simulink model "test_case_generation_SOC"  (R2015b)
settings: Solver=FixedStepDiscrete  StartTime=0.0  StopTime=final_time  FixedStep=0.1  RelTol=1e-3
values from neighbouring files (symbols this model uses):
  BMSk_stepSize = 0.1    [soc_test_case_init.m]
  cell_ocvs_sampling = sampling_time    (= 0.1)    [soc_test_case_init.m]
  cell_socs_sampling = sampling_time    (= 0.1)    [soc_test_case_init.m]
  cell_temps_sampling = sampling_time    (= 0.1)    [soc_test_case_init.m]
  cell_voltages_sampling = sampling_time    (= 0.1)    [soc_test_case_init.m]
  charge_cycle = 4    [soc_test_case_init.m]
  inital_outlet_temperature = air_temperature    (= 35)    [soc_test_case_init.m]
  initial_cell_ocvs = Initial_Volt*ones(NUM_CELL_SERIES,1)    [soc_test_case_init.m]
  initial_cell_socs = Initial_SOC*ones(NUM_CELL_SERIES,1)    [soc_test_case_init.m]
  initial_cell_temps = air_temperature*ones(NUM_CELL_SERIES,1)    [soc_test_case_init.m]
  initial_cell_voltages = Initial_Volt*ones(NUM_CELL_SERIES,1)    [soc_test_case_init.m]
  initial_pack_current = 0    [soc_test_case_init.m]
  initial_pack_soc = Initial_SOC    (= 79)    [soc_test_case_init.m]
  initial_pack_voltage = 161    [soc_test_case_init.m]
  initial_vehicle_side_voltage = 0    [soc_test_case_init.m]
  pack_current_sampling = sampling_time    (= 0.1)    [soc_test_case_init.m]
  pack_soc_sampling = sampling_time    (= 0.1)    [soc_test_case_init.m]
  pack_voltage_sampling = sampling_time    (= 0.1)    [soc_test_case_init.m]
  vehicle_side_voltage_sampling = sampling_time    (= 0.1)    [soc_test_case_init.m]
undefined symbols (not defined in the file or in its folder): sigbuilder_block
libraries: simulink x4
(part 1 of 2)
settings Model: Creator=nctzv8  LastModifiedBy=nctzv8
settings ConfigSet: Description=OpenECU configuration set for code generation under RTW-EC.
settings SolverCC: PositivePriorityOrder=on
settings DataIOCC: SaveFormat=Array  SignalLoggingSaveFormat=ModelDataLogs
settings OptimizationCC: DefaultParameterBehavior=Inlined  InlineInvariantSignals=on  ExpressionDepthLimit=2147483647  StateBitsets=on  DataBitsets=on  ZeroExternalMemoryAtStartup=off  ZeroInternalMemoryAtStartup=off  NoFixptDivByZeroProtection=on  EfficientFloat2IntCast=on  OptimizeModelRefInitCode=on  LifeSpan=1
settings DebuggingCC: SaveWithParameterizedLinksMsg=none  UnderspecifiedInitializationDetection=Classic  MergeDetectMultiDrivingBlocksExec=none  SignalResolutionControl=TryResolveAllWithWarning  MultiTaskDSMMsg=warning  MultiTaskCondExecSysMsg=none  SingleTaskRateTransMsg=error  CheckMatrixSingularityMsg=warning  VectorMatrixConversionMsg=warning  FcnCallInpInsideContextMsg=UseLocalSettings  SignalLabelMismatchMsg=warning  StateNameClashWarn=warning
settings HardwareCC: ProdBitPerPointer=32  ProdLargestAtomicInteger=Long  ProdLargestAtomicFloat=Double  ProdEndianess=BigEndian  ProdWordSize=32  ProdHWDeviceType=Freescale->32-bit PowerPC  TargetIntDivRoundTo=Zero  TargetEndianess=BigEndian  TargetHWDeviceType=Freescale->32-bit PowerPC  ProdEqTarget=off
settings RTWCC: SystemTargetFile=openecu_ert.tlc  MakeCommand=make_rtw optimized_floating_point=1  TemplateMakefile=openecu_ert_r2015b_64.tmf  Description=OpenECU Platform Target (ERT, optimised floating-point code)  RetainRTWFile=on  IncludeHyperlinkInReport=on
settings CodeAppCC: ForceParamTrailComments=on  IgnoreCustomStorageClasses=off  SimulinkDataObjDesc=on  CustomSymbolStrType=$N$R$M  InsertBlockDesc=on  InternalIdentifier=Classic
settings STFCustomTargetCC: TargetLibSuffix=.a  GenerateSampleERTMain=on  ConcurrentExecutionCompliant=off  IncludeMdlTerminateFcn=off  GeneratePreprocessorConditionals=Use local settings  CombineOutputUpdateFcns=on  IncludeFileDelimiter=UseQuote  ERTCustomFileBanners=on  SupportContinuousTime=off  MATLABClassNameForMDSCustomization=Simulink.SoftwareTarget.ERTCustomization  CPPClassGenCompliant=off  GRTInterface=off  SystemTargetFile=openecu_ert.tlc
settings ERTTargetCC: GenerateSampleERTMain=on  ParMdlRefBuildCompliant=off  CompOptLevelCompliant=off  ConcurrentExecutionCompliant=off  IncludeMdlTerminateFcn=off  ERTFirstTimeCompliant=off  IncludeFileDelimiter=UseQuote  SupportNonInlinedSFcns=on  ModelStepFunctionPrototypeControlCompliant=off  CPPClassGenCompliant=off  UseToolchainInfoCompliant=off  ExtModeMexFile=noextcomm  InlinedParameterPlacement=NonHierarchical  ERTSrcFileBannerTemplate=oe_code_c_template.cgt  ERTHdrFileBannerTemplate=oe_code_h_template.cgt  ERTDataSrcFileTemplate=oe_data_c_template.cgt  ERTDataHdrFileTemplate=oe_data_h_template.cgt  ERTCustomFileTemplate=example_file_process.tlc  GlobalDataDefinition=InSeparateSourceFile  GlobalDataReference=InSeparateHeaderFile  EnableUserReplacementTypes=on

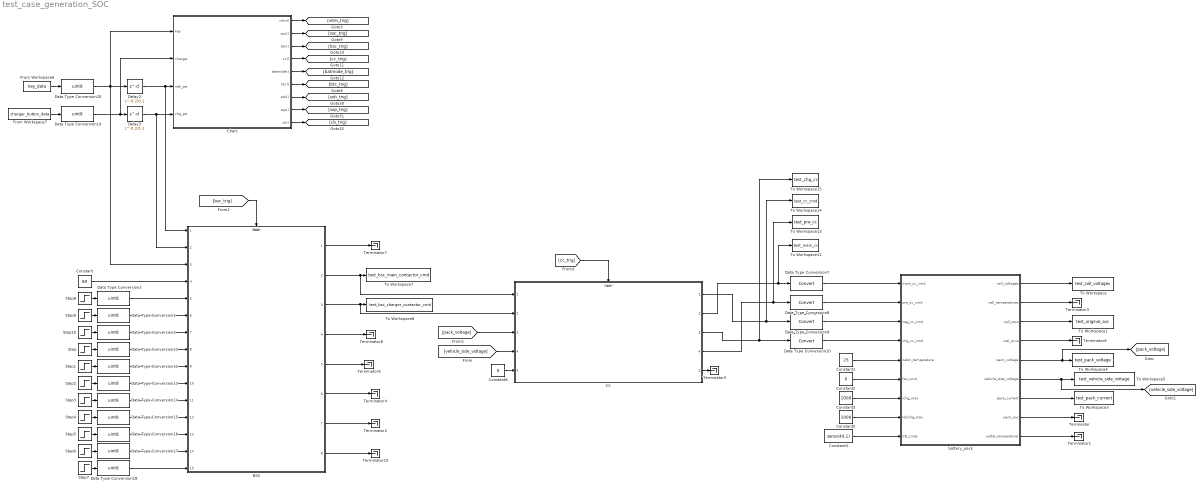
== system test_case_generation_SOC ==
  BSC : ModelReference  ModelNameDialog=BSC.slx  SimulationMode=Normal  ModelReferenceVersion=1.220  CopyOfModelName=BSC.slx  TriggerPortName=Trigger  TriggerPortTriggerType=function-call  TriggerPortStatesWhenEnabling=held
  CC : ModelReference  ModelNameDialog=CC.slx  SimulationMode=Normal  ModelReferenceVersion=1.108  CopyOfModelName=CC.slx  TriggerPortName=Trigger  TriggerPortTriggerType=function-call  TriggerPortStatesWhenEnabling=held
  Chart : Stateflow chart  TreatAsAtomicUnit=on
  Constant : Constant  Value=80
  Constant1 : Constant  Value=25
  Constant2 : Constant  Value=0
  Constant3 : Constant  Value=1000
  Constant4 : Constant  Value=zeros(40,1)
  Constant5 : Constant  Value=1000
  Constant6 : Constant  Value=0
  Data Type Conversion{1..3,11..20} (13 alike) : DataTypeConversion  OutDataTypeStr=uint8
  Data Type Conversion{7..10} (4 alike) : DataTypeConversion
  Delay2 : Delay  DelayLength=0.2/0.1
  Delay3 : Delay  DelayLength=0.2/0.1
  From Workspace6 : FromWorkspace  VariableName=key_data
  From Workspace7 : FromWorkspace  VariableName=charger_button_data
  Step{,1..10} (11 alike) : Step  Time=0  After=0  VectorParams1D=off
  Terminator{,1..10} (11 alike) : Terminator
  To Workspace : ToWorkspace  VariableName=test_cell_voltages  SaveFormat=Timeseries  SampleTime=-1
  To Workspace1 : ToWorkspace  VariableName=test_original_soc  SaveFormat=Timeseries  SampleTime=-1
  To Workspace12 : ToWorkspace  VariableName=test_main_cc  SaveFormat=Timeseries  SampleTime=-1
  To Workspace13 : ToWorkspace  VariableName=test_pre_cc  SaveFormat=Timeseries  SampleTime=-1
  To Workspace14 : ToWorkspace  VariableName=test_cc_cmd  SaveFormat=Timeseries  SampleTime=-1
  To Workspace15 : ToWorkspace  VariableName=test_chg_cc  SaveFormat=Timeseries  SampleTime=-1
  To Workspace3 : ToWorkspace  VariableName=test_pack_current  SaveFormat=Timeseries  SampleTime=-1
  To Workspace4 : ToWorkspace  VariableName=test_pack_voltage  SaveFormat=Timeseries  SampleTime=-1
  To Workspace5 : ToWorkspace  VariableName=test_vehicle_side_voltage  SaveFormat=Timeseries  SampleTime=-1
  To Workspace7 : ToWorkspace  VariableName=test_bsc_main_contactor_cmd  SaveFormat=Timeseries  SampleTime=-1
  To Workspace8 : ToWorkspace  VariableName=test_bsc_charger_contactor_cmd  SaveFormat=Timeseries  SampleTime=-1
  battery_pack : Subsystem
  wires:
  battery_pack/1(cell_voltages) -> To Workspace/1
  battery_pack/2(cell_temperatures) -> Terminator3/1
  battery_pack/3(cell_socs) -> To Workspace1/1
  battery_pack/4(cell_ocvs) -> Terminator6/1
  battery_pack/5(pack_voltage) -> [pack_voltage], To Workspace4/1
  battery_pack/6(vehicle_side_voltage) -> [vehicle_side_voltage], To Workspace5/1
  battery_pack/7(pack_current) -> To Workspace3/1
  battery_pack/8(pack_soc) -> Terminator/1
  battery_pack/9(outlet_temperature) -> Terminator1/1
  Constant1/1 -> battery_pack/5(cabin_temperature)
  Constant2/1 -> battery_pack/6(fan_cmd)
  Constant3/1 -> battery_pack/7(Ichg_max)
  Constant4/1 -> battery_pack/9(CB_cmds)
  Constant5/1 -> battery_pack/8(Idischg_max)
  Data Type Conversion7/1 -> battery_pack/1(main_cc_cmd)
  Data Type Conversion8/1 -> battery_pack/2(pre_cc_cmd)
  Data Type Conversion10/1 -> battery_pack/4(chg_cc_cmd)
  CC/1 -> To Workspace14/1, Data Type Conversion9/1
  CC/2 -> To Workspace12/1, Data Type Conversion7/1
  CC/3 -> To Workspace15/1, Data Type Conversion10/1
  CC/4 -> To Workspace13/1, Data Type Conversion8/1
  Constant/1 -> BSC/4
  Data Type Conversion2/1 -> BSC/5
  Data Type Conversion1/1 -> BSC/6
  Data Type Conversion3/1 -> BSC/7
  Data Type Conversion12/1 -> BSC/8
  Data Type Conversion13/1 -> BSC/10
  Data Type Conversion11/1 -> BSC/9
  Data Type Conversion14/1 -> BSC/11
  Data Type Conversion15/1 -> BSC/12
  Data Type Conversion17/1 -> BSC/14
  Data Type Conversion18/1 -> BSC/15
  Data Type Conversion16/1 -> BSC/13
  [bsc_trig] -> BSC/Trigger
  BSC/1 -> Terminator7/1
  BSC/2 -> CC/1, To Workspace7/1
  BSC/3 -> CC/2, To Workspace8/1
  BSC/4 -> Terminator8/1
  BSC/5 -> Terminator9/1
  BSC/7 -> Terminator2/1
  BSC/6 -> Terminator4/1
  BSC/8 -> Terminator10/1
  [vehicle_side_voltage] -> CC/4
  [pack_voltage] -> CC/3
  Constant6/1 -> CC/5
  [cc_trig] -> CC/Trigger
  Data Type Conversion9/1 -> battery_pack/3(neg_cc_cmd)
  CC/5 -> Terminator5/1
  Step2/1 -> Data Type Conversion13/1
  Step1/1 -> Data Type Conversion11/1
  Step3/1 -> Data Type Conversion14/1
  Step4/1 -> Data Type Conversion15/1
  Step6/1 -> Data Type Conversion17/1
  Step7/1 -> Data Type Conversion18/1
  Step5/1 -> Data Type Conversion16/1
  Step/1 -> Data Type Conversion12/1
  Step10/1 -> Data Type Conversion3/1
  Step9/1 -> Data Type Conversion1/1
  Step8/1 -> Data Type Conversion2/1
  Chart/1(vitm()) -> [vitm_trig]
  Chart/2(soc()) -> [soc_trig]
  Chart/3(bsc()) -> [bsc_trig]
  Chart/4(cc()) -> [cc_trig]
  Chart/5(batmode()) -> [batmode_trig]
  Chart/6(btc()) -> [btc_trig]
  Delay2/1 -> BSC/1, Chart/3(veh_psr)
  Chart/7(soh()) -> [soh_trig]
  Chart/8(sop()) -> [sop_trig]
  Chart/9(cb()) -> [cb_trig]
  Delay3/1 -> BSC/2, Chart/4(chg_psr)
  Data Type Conversion19/1 -> Chart/2(charger), Delay3/1
  Data Type Conversion20/1 -> BSC/3, Chart/1(key), Delay2/1
  From Workspace6/1 -> Data Type Conversion20/1
  From Workspace7/1 -> Data Type Conversion19/1

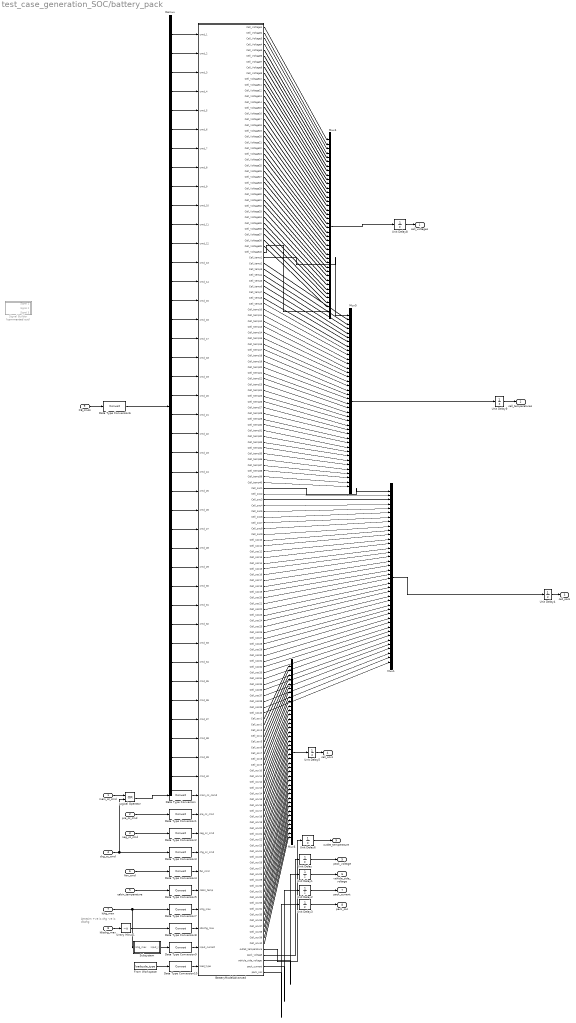
== system test_case_generation_SOC/battery_pack ==
  note: Amesim
      | +ve is chg
      | -ve is dischg
  main_cc_cmd : Inport
  pre_cc_cmd : Inport  Port=2
  neg_cc_cmd : Inport  Port=3
  chg_cc_cmd : Inport  Port=4
  cabin_temperature : Inport  Port=5
  fan_cmd : Inport  Port=6
  Ichg_max : Inport  Port=7
  Idischg_max : Inport  Port=8
  CB_cmds : Inport  Port=9
  BatteryModelAdvanced : Subsystem  Tag=AME2SLCoSim  InitFcn=AMESimLib_initBlock  StartFcn=AMESimLib_startBlock  StopFcn=AMESimLib_stopBlock
      settings: DeleteFcn=AMESimLib_deleteBlock  OpenFcn=AMESimLib_openBlock('AME2SLCoSim')
      mask Display: image(imread('amesim_pix256.png'),[0.4,0.7,0.2,0.2]);disp('Simcenter Amesim co-Sim:\nBatteryModelAdvanced');port_label('input',1,'cmd_1');port_label('input',2,'cmd_2');port_label('input',3,'cmd_3');port_label('input',4,'cmd_4');port_label('input',5,'cmd_5');port_label('input',6,'cmd_6');port_label('input',7,'cmd_7');port_label('input',8,'cmd_8');port_label('input',9,'cmd_9');port_label('input',10,'cmd_10');port_label('input',11,'cmd_11');port_label('input',12,'cmd_12');port_label('input',13,'cmd_13');port_label('input',14,'cmd_14');port_label('input',15,'cmd_15');port_label('input',16,'cmd_16');port_label('input',17,'cmd_17');port_label('input',18,'cmd_18');port_label('input',19,'cmd_19');port_label('input',20,'cmd_20');port_label('input',21,'cmd_21');port_label('input',22,'cmd_22');port_label('input',23,'cmd_23');port_label('input',24,'cmd_24');port_label('input',25,'cmd_25');port_label('input',26,'cmd_26');port_label('input',27,'cmd_27');port_label('input',28,'cmd_28');port_label('input',29,'cmd_29');port_label('input',30,'cmd_30');port_label('input',31,'cmd_31');port_label('input',32,'cmd_32');port_label('input',33,'cmd_33');port_label('input',34,'cmd_34');port_label('input',35,'cmd_35');port_label('input',36,'cmd_36');port_label('input',37,'cmd_37');port_label('input',38,'cmd_38');port_label('input',39,'cmd_39');port_label('input',40,'cmd_40');port_label('input',41,'main_cc_comd');port_label('input',42,'pre_cc_cmd');port_label('input',43,'neg_cc_cmd');port_label('input',44,'chg_cc_cmd');port_label('input',45,'fan_cmd');port_label('input',46,'cabin_temp');port_label('input',47,'Ichg_max');port_label('input',48,'Idischg_max');port_label('input',49,'input_current');port_label('input',50,'load_type');port_label('output',1,'Cell_Voltage1');port_label('output',2,'Cell_Voltage2');port_label('output',3,'Cell_Voltage3');port_label('output',4,'Cell_Voltage4');port_label('output',5,'Cell_Voltage5');port_label('output',6,'Cell_Voltage6');port_label('output',7,'Cell_Voltage7');port_label('output',8,'Cell_Voltage8');port_label('output',9,'Cell_Voltage9');port_label('output',10,'Cell_Voltage10');port_label('output',11,'Cell_Voltage11');port_label('output',12,'Cell_Voltage12');port_label('output',13,'Cell_Voltage13');port_label('output',14,'Cell_Voltage14');port_label('output',15,'Cell_Voltage15');port_label('output',16,'Cell_Voltage16');port_label('output',17,'Cell_Voltage17');port_label('output',18,'Cell_Voltage18');port_label('output',19,'Cell_Voltage19');port_label('output',20,'Cell_Voltage20');port_label('output',21,'Cell_Voltage21');port_label('output',22,'Cell_Voltage22');port_label('output',23,'Cell_Voltage23');port_label('output',24,'Cell_Voltage24');port_label('output',25,'Cell_Voltage25');port_label('output',26,'Cell_Voltage26');port_label('output',27,'Cell_Voltage27');port_label('output',28,'Cell_Voltage28');port_label('output',29,'Cell_Voltage29');port_label('output',30,'Cell_Voltage30');port_label('output',31,'Cell_Voltage31');port_label('output',32,'Cell_Voltage32');port_label('output',33,'Cell_Voltage33');port_label('output',34,'Cell_Voltage34');port_label('output',35,'Cell_Voltage35');port_label('output',36,'Cell_Voltage36');port_label('output',37,'Cell_Voltage37');port_label('output',38,'Cell_Voltage38');port_label('output',39,'Cell_Voltage39');port_label('output',40,'Cell_Voltage40');port_label('output',41,'Cell_temp1');port_label('output',42,'Cell_temp2');port_label('output',43,'Cell_temp3');port_label('output',44,'Cell_temp4');port_label('output',45,'Cell_temp5');port_label('output',46,'Cell_temp6');port_label('output',47,'Cell_temp7');port_label('output',48,'Cell_temp8');port_label('output',49,'Cell_temp9');port_label('output',50,'Cell_temp10');port_label('output',51,'Cell_temp11');port_label('output',52,'Cell_temp12');port_label('output',53,'Cell_temp13');port_label('output',54,'Cell_temp14');port_label('output',55,'Cell_temp15');port_label('output',56,'Cell_temp16');port_label('output',57,'Cell_temp17');port_label('output',58,'Cell_temp18');port_label('output',59,'Cell_temp19');port_label('output',60,'Cell_temp20');port_label('output',61,'Cell_temp21');port_label('output',62,'Cell_temp22');port_label('output',63,'Cell_temp23');port_label('output',64,'Cell_temp24');port_label('output',65,'Cell_temp25');port_label('output',66,'Cell_temp26');port_label('output',67,'Cell_temp27');port_label('output',68,'Cell_temp28');port_label('output',69,'Cell_temp29');port_label('output',70,'Cell_temp30');port_label('output',71,'Cell_temp31');port_label('output',72,'Cell_temp32');port_label('output',73,'Cell_temp33');port_label('output',74,'Cell_temp34');port_label('output',75,'Cell_temp35');port_label('output',76,'Cell_temp36');port_label('output',77,'Cell_temp37');port_label('output',78,'Cell_temp38');port_label('output',79,'Cell_temp39');port_label('output',80,'Cell_temp40');port_label('output',81,'Cell_soc1');port_label('output',82,'Cell_soc2');port_label('output',83,'Cell_soc3');port_label('output',84,'Cell_soc4');port_label('output',85,'Cell_soc5');port_label('output',86,'Cell_soc6');port_label('output',87,'Cell_soc7');port_label('output',88,'Cell_soc8');port_label('output',89,'Cell_soc9');port_label('output',90,'Cell_soc10');port_label('output',91,'Cell_soc11');port_label('output',92,'Cell_soc12');port_label('output',93,'Cell_soc13');port_label('output',94,'Cell_soc14');port_label('output',95,'Cell_soc15');port_label('output',96,'Cell_soc16');port_label('output',97,'Cell_soc17');port_label('output',98,'Cell_soc18');port_label('output',99,'Cell_soc19');port_label('output',100,'Cell_soc20');port_label('output',101,'Cell_soc21');port_label('output',102,'Cell_soc22');port_label('output',103,'Cell_soc23');port_label('output',104,'Cell_soc24');port_label('output',105,'Cell_soc25');port_label('output',106,'Cell_soc26');port_label('output',107,'Cell_soc27');port_label('output',108,'Cell_soc28');port_label('output',109,'Cell_soc29');port_label('output',110,'Cell_soc30');port_label('output',111,'Cell_soc31');port_label('output',112,'Cell_soc32');port_label('output',113,'Cell_soc33');port_label('output',114,'Cell_soc34');port_label('output',115,'Cell_soc35');port_label('output',116,'Cell_soc36');port_label('output',117,'Cell_soc37');port_label('output',118,'Cell_soc38');port_label('output',119,'Cell_soc39');port_label('output',120,'Cell_soc40');port_label('output',121,'Cell_ocv1');port_label('output',122,'Cell_ocv2');port_label('output',123,'Cell_ocv3');port_label('output',124,'Cell_ocv4');port_label('output',125,'Cell_ocv5');port_label('output',126,'Cell_ocv6');port_label('output',127,'Cell_ocv7');port_label('output',128,'Cell_ocv8');port_label('output',129,'Cell_ocv9');port_label('output',130,'Cell_ocv10');port_label('output',131,'Cell_ocv11');port_label('output',132,'Cell_ocv12');port_label('output',133,'Cell_ocv13');port_label('output',134,'Cell_ocv14');port_label('output',135,'Cell_ocv15');port_label('output',136,'Cell_ocv16');port_label('output',137,'Cell_ocv17');port_label('output',138,'Cell_ocv18');port_label('output',139,'Cell_ocv19');port_label('output',140,'Cell_ocv20');port_label('output',141,'Cell_ocv21');port_label('output',142,'Cell_ocv22');port_label('output',143,'Cell_ocv23');port_label('output',144,'Cell_ocv24');port_label('output',145,'Cell_ocv25');port_label('output',146,'Cell_ocv26');port_label('output',147,'Cell_ocv27');port_label('output',148,'Cell_ocv28');port_label('output',149,'Cell_ocv29');port_label('output',150,'Cell_ocv30');port_label('output',151,'Cell_ocv31');port_label('output',152,'Cell_ocv32');port_label('output',153,'Cell_ocv33');port_label('output',154,'Cell_ocv34');port_label('output',155,'Cell_ocv35');port_label('output',156,'Cell_ocv36');port_label('output',157,'Cell_ocv37');port_label('output',158,'Cell_ocv38');port_label('output',159,'Cell_ocv39');port_label('output',160,'Cell_ocv40');port_label('output',161,'outlet_temperature');port_label('output',162,'pack_voltage');port_label('output',163,'vehicle_side_voltage');port_label('output',164,'pack_current');port_label('output',165,'pack_soc');
  Data Type Conversion{,1..10} (11 alike) : DataTypeConversion
  Demux : Demux  Outputs=40
  From Workspace : FromWorkspace  VariableName=loadcycle_type
  Logical Operator : Logic  Operator=OR  AllPortsSameDT=off  OutDataTypeStr=boolean
  Mux{1,4..6} (4 alike) : Mux  Inputs=40
  Signal Builder : Subsystem  Tag=STV Subsys  Commented=on  LoadFcn=sigbuilder_block('load');  StartFcn=sigbuilder_block('start');  StopFcn=sigbuilder_block('stop');  ClipboardFcn=sigbuilder_block('clipboard');  mask(Sigbuilder block){}
      mask help: Simulink:masks:SigbuilderBlock_MD
      mask init:
      | if ~strcmp(get_param(bdroot(gcbh),'SimulationStatus'),'stopped') tuvar = sigbuilder_block('maskInit'); end
      settings: CopyFcn=sigbuilder_block('copy');  DeleteFcn=sigbuilder_block('delete');  ModelCloseFcn=sigbuilder_block('modelClose');  PreSaveFcn=sigbuilder_block('preSave');  PauseFcn=sigbuilder_block('pause');  ContinueFcn=sigbuilder_block('continue');  NameChangeFcn=sigbuilder_block('namechange');  OpenFcn=sigbuilder_block('open',[5.4 5.4 1141.2 580.8 ]);  CloseFcn=sigbuilder_block('close');
      mask Display: plot(0, 0, 100, 100,[2, 2, 32, 32, 2], [68, 8, 8, 68, 68],[32, 2], [38, 38], [32, 19, 2],[53, 60, 44], [32, 17, 17, 2],[16, 16, 31, 31]);txt = getActiveGroup(gcbh);text(2, 100, txt,'verticalAlignment', 'top');
  Subsystem : Subsystem
  Unary Minus1 : UnaryMinus
  Unit Delay : UnitDelay  InitialCondition=initial_pack_voltage  SampleTime=pack_voltage_sampling
  Unit Delay1 : UnitDelay  InitialCondition=initial_vehicle_side_voltage  SampleTime=vehicle_side_voltage_sampling
  Unit Delay2 : UnitDelay  InitialCondition=initial_pack_current  SampleTime=pack_current_sampling
  Unit Delay3 : UnitDelay  InitialCondition=initial_pack_soc  SampleTime=pack_soc_sampling
  Unit Delay4 : UnitDelay  InitialCondition=initial_cell_socs  SampleTime=cell_socs_sampling
  Unit Delay5 : UnitDelay  InitialCondition=initial_cell_ocvs  SampleTime=cell_ocvs_sampling
  Unit Delay6 : UnitDelay  InitialCondition=inital_outlet_temperature  SampleTime=pack_voltage_sampling
  Unit Delay8 : UnitDelay  InitialCondition=initial_cell_voltages  SampleTime=cell_voltages_sampling
  Unit Delay9 : UnitDelay  InitialCondition=initial_cell_temps  SampleTime=cell_temps_sampling
  cell_voltages : Outport
  cell_temperatures : Outport  Port=2
  cell_socs : Outport  Port=3
  cell_ocvs : Outport  Port=4
  pack_voltage : Outport  Port=5
  vehicle_side_voltage : Outport  Port=6
  pack_current : Outport  Port=7
  pack_soc : Outport  Port=8
  outlet_temperature : Outport  Port=9
  wires:
  Unit Delay/1 -> pack_voltage/1
  Unit Delay1/1 -> vehicle_side_voltage/1
  Unit Delay2/1 -> pack_current/1
  Unit Delay3/1 -> pack_soc/1
  Unit Delay8/1 -> cell_voltages/1
  Mux4/1 -> Unit Delay8/1
  Mux5/1 -> Unit Delay9/1
  Unit Delay9/1 -> cell_temperatures/1
  Mux1/1 -> Unit Delay4/1
  Unit Delay4/1 -> cell_socs/1
  Mux6/1 -> Unit Delay5/1
  Unit Delay5/1 -> cell_ocvs/1
  BatteryModelAdvanced/41(Cell_temp1) -> Mux5/1
  BatteryModelAdvanced/42(Cell_temp2) -> Mux5/2
  BatteryModelAdvanced/43(Cell_temp3) -> Mux5/3
  BatteryModelAdvanced/44(Cell_temp4) -> Mux5/4
  BatteryModelAdvanced/45(Cell_temp5) -> Mux5/5
  BatteryModelAdvanced/46(Cell_temp6) -> Mux5/6
  BatteryModelAdvanced/47(Cell_temp7) -> Mux5/7
  BatteryModelAdvanced/48(Cell_temp8) -> Mux5/8
  BatteryModelAdvanced/49(Cell_temp9) -> Mux5/9
  BatteryModelAdvanced/50(Cell_temp10) -> Mux5/10
  BatteryModelAdvanced/51(Cell_temp11) -> Mux5/11
  BatteryModelAdvanced/52(Cell_temp12) -> Mux5/12
  BatteryModelAdvanced/53(Cell_temp13) -> Mux5/13
  BatteryModelAdvanced/54(Cell_temp14) -> Mux5/14
  BatteryModelAdvanced/55(Cell_temp15) -> Mux5/15
  BatteryModelAdvanced/56(Cell_temp16) -> Mux5/16
  BatteryModelAdvanced/57(Cell_temp17) -> Mux5/17
  BatteryModelAdvanced/58(Cell_temp18) -> Mux5/18
  BatteryModelAdvanced/59(Cell_temp19) -> Mux5/19
  BatteryModelAdvanced/60(Cell_temp20) -> Mux5/20
  BatteryModelAdvanced/61(Cell_temp21) -> Mux5/21
  BatteryModelAdvanced/62(Cell_temp22) -> Mux5/22
  BatteryModelAdvanced/63(Cell_temp23) -> Mux5/23
  BatteryModelAdvanced/64(Cell_temp24) -> Mux5/24
  BatteryModelAdvanced/65(Cell_temp25) -> Mux5/25
  BatteryModelAdvanced/66(Cell_temp26) -> Mux5/26
  BatteryModelAdvanced/67(Cell_temp27) -> Mux5/27
  BatteryModelAdvanced/68(Cell_temp28) -> Mux5/28
  BatteryModelAdvanced/69(Cell_temp29) -> Mux5/29
  BatteryModelAdvanced/70(Cell_temp30) -> Mux5/30
  BatteryModelAdvanced/71(Cell_temp31) -> Mux5/31
  BatteryModelAdvanced/72(Cell_temp32) -> Mux5/32
  BatteryModelAdvanced/73(Cell_temp33) -> Mux5/33
  BatteryModelAdvanced/74(Cell_temp34) -> Mux5/34
  BatteryModelAdvanced/75(Cell_temp35) -> Mux5/35
  BatteryModelAdvanced/76(Cell_temp36) -> Mux5/36
  BatteryModelAdvanced/77(Cell_temp37) -> Mux5/37
  BatteryModelAdvanced/78(Cell_temp38) -> Mux5/38
  BatteryModelAdvanced/79(Cell_temp39) -> Mux5/39
  BatteryModelAdvanced/80(Cell_temp40) -> Mux5/40
  BatteryModelAdvanced/1(Cell_Voltage1) -> Mux4/1
  BatteryModelAdvanced/2(Cell_Voltage2) -> Mux4/2
  BatteryModelAdvanced/3(Cell_Voltage3) -> Mux4/3
  BatteryModelAdvanced/4(Cell_Voltage4) -> Mux4/4
  BatteryModelAdvanced/5(Cell_Voltage5) -> Mux4/5
  BatteryModelAdvanced/6(Cell_Voltage6) -> Mux4/6
  BatteryModelAdvanced/7(Cell_Voltage7) -> Mux4/7
  BatteryModelAdvanced/8(Cell_Voltage8) -> Mux4/8
  BatteryModelAdvanced/9(Cell_Voltage9) -> Mux4/9
  BatteryModelAdvanced/10(Cell_Voltage10) -> Mux4/10
  BatteryModelAdvanced/11(Cell_Voltage11) -> Mux4/11
  BatteryModelAdvanced/12(Cell_Voltage12) -> Mux4/12
  BatteryModelAdvanced/13(Cell_Voltage13) -> Mux4/13
  BatteryModelAdvanced/14(Cell_Voltage14) -> Mux4/14
  BatteryModelAdvanced/15(Cell_Voltage15) -> Mux4/15
  BatteryModelAdvanced/16(Cell_Voltage16) -> Mux4/16
  BatteryModelAdvanced/17(Cell_Voltage17) -> Mux4/17
  BatteryModelAdvanced/18(Cell_Voltage18) -> Mux4/18
  BatteryModelAdvanced/19(Cell_Voltage19) -> Mux4/19
  BatteryModelAdvanced/20(Cell_Voltage20) -> Mux4/20
  BatteryModelAdvanced/21(Cell_Voltage21) -> Mux4/21
  BatteryModelAdvanced/22(Cell_Voltage22) -> Mux4/22
  BatteryModelAdvanced/23(Cell_Voltage23) -> Mux4/23
  BatteryModelAdvanced/24(Cell_Voltage24) -> Mux4/24
  BatteryModelAdvanced/25(Cell_Voltage25) -> Mux4/25
  BatteryModelAdvanced/26(Cell_Voltage26) -> Mux4/26
  BatteryModelAdvanced/27(Cell_Voltage27) -> Mux4/27
  BatteryModelAdvanced/28(Cell_Voltage28) -> Mux4/28
  BatteryModelAdvanced/29(Cell_Voltage29) -> Mux4/29
  BatteryModelAdvanced/30(Cell_Voltage30) -> Mux4/30
  BatteryModelAdvanced/31(Cell_Voltage31) -> Mux4/31
  BatteryModelAdvanced/32(Cell_Voltage32) -> Mux4/32
  BatteryModelAdvanced/33(Cell_Voltage33) -> Mux4/33
  BatteryModelAdvanced/34(Cell_Voltage34) -> Mux4/34
  BatteryModelAdvanced/35(Cell_Voltage35) -> Mux4/35
  BatteryModelAdvanced/36(Cell_Voltage36) -> Mux4/36
  BatteryModelAdvanced/37(Cell_Voltage37) -> Mux4/37
  BatteryModelAdvanced/38(Cell_Voltage38) -> Mux4/38
  BatteryModelAdvanced/39(Cell_Voltage39) -> Mux4/39
  BatteryModelAdvanced/40(Cell_Voltage40) -> Mux4/40
  BatteryModelAdvanced/81(Cell_soc1) -> Mux1/1
  BatteryModelAdvanced/82(Cell_soc2) -> Mux1/2
  BatteryModelAdvanced/83(Cell_soc3) -> Mux1/3
  BatteryModelAdvanced/84(Cell_soc4) -> Mux1/4
  BatteryModelAdvanced/85(Cell_soc5) -> Mux1/5
  BatteryModelAdvanced/86(Cell_soc6) -> Mux1/6
  BatteryModelAdvanced/87(Cell_soc7) -> Mux1/7
  BatteryModelAdvanced/88(Cell_soc8) -> Mux1/8
  BatteryModelAdvanced/89(Cell_soc9) -> Mux1/9
  BatteryModelAdvanced/90(Cell_soc10) -> Mux1/10
  BatteryModelAdvanced/91(Cell_soc11) -> Mux1/11
  BatteryModelAdvanced/92(Cell_soc12) -> Mux1/12
  BatteryModelAdvanced/93(Cell_soc13) -> Mux1/13
  BatteryModelAdvanced/94(Cell_soc14) -> Mux1/14
  BatteryModelAdvanced/95(Cell_soc15) -> Mux1/15
  BatteryModelAdvanced/96(Cell_soc16) -> Mux1/16
  BatteryModelAdvanced/97(Cell_soc17) -> Mux1/17
  BatteryModelAdvanced/98(Cell_soc18) -> Mux1/18
  BatteryModelAdvanced/99(Cell_soc19) -> Mux1/19
  BatteryModelAdvanced/100(Cell_soc20) -> Mux1/20
  BatteryModelAdvanced/101(Cell_soc21) -> Mux1/21
  BatteryModelAdvanced/102(Cell_soc22) -> Mux1/22
  BatteryModelAdvanced/103(Cell_soc23) -> Mux1/23
  BatteryModelAdvanced/104(Cell_soc24) -> Mux1/24
  BatteryModelAdvanced/105(Cell_soc25) -> Mux1/25
  BatteryModelAdvanced/106(Cell_soc26) -> Mux1/26
  BatteryModelAdvanced/107(Cell_soc27) -> Mux1/27
  BatteryModelAdvanced/108(Cell_soc28) -> Mux1/28
  BatteryModelAdvanced/109(Cell_soc29) -> Mux1/29
  BatteryModelAdvanced/110(Cell_soc30) -> Mux1/30
  BatteryModelAdvanced/111(Cell_soc31) -> Mux1/31
  BatteryModelAdvanced/112(Cell_soc32) -> Mux1/32
  BatteryModelAdvanced/113(Cell_soc33) -> Mux1/33
  BatteryModelAdvanced/114(Cell_soc34) -> Mux1/34
  BatteryModelAdvanced/115(Cell_soc35) -> Mux1/35
  BatteryModelAdvanced/116(Cell_soc36) -> Mux1/36
  BatteryModelAdvanced/117(Cell_soc37) -> Mux1/37
  BatteryModelAdvanced/118(Cell_soc38) -> Mux1/38
  BatteryModelAdvanced/119(Cell_soc39) -> Mux1/39
  BatteryModelAdvanced/120(Cell_soc40) -> Mux1/40
  BatteryModelAdvanced/121(Cell_ocv1) -> Mux6/1
  BatteryModelAdvanced/122(Cell_ocv2) -> Mux6/2
  BatteryModelAdvanced/123(Cell_ocv3) -> Mux6/3
  BatteryModelAdvanced/124(Cell_ocv4) -> Mux6/4
  BatteryModelAdvanced/125(Cell_ocv5) -> Mux6/5
  BatteryModelAdvanced/126(Cell_ocv6) -> Mux6/6
  BatteryModelAdvanced/127(Cell_ocv7) -> Mux6/7
  BatteryModelAdvanced/128(Cell_ocv8) -> Mux6/8
  BatteryModelAdvanced/129(Cell_ocv9) -> Mux6/9
  BatteryModelAdvanced/130(Cell_ocv10) -> Mux6/10
  BatteryModelAdvanced/131(Cell_ocv11) -> Mux6/11
  BatteryModelAdvanced/132(Cell_ocv12) -> Mux6/12
  BatteryModelAdvanced/133(Cell_ocv13) -> Mux6/13
  BatteryModelAdvanced/134(Cell_ocv14) -> Mux6/14
  BatteryModelAdvanced/135(Cell_ocv15) -> Mux6/15
  BatteryModelAdvanced/136(Cell_ocv16) -> Mux6/16
  BatteryModelAdvanced/137(Cell_ocv17) -> Mux6/17
  BatteryModelAdvanced/138(Cell_ocv18) -> Mux6/18
  BatteryModelAdvanced/139(Cell_ocv19) -> Mux6/19
  BatteryModelAdvanced/140(Cell_ocv20) -> Mux6/20
  BatteryModelAdvanced/141(Cell_ocv21) -> Mux6/21
  BatteryModelAdvanced/142(Cell_ocv22) -> Mux6/22
  BatteryModelAdvanced/143(Cell_ocv23) -> Mux6/23
  BatteryModelAdvanced/144(Cell_ocv24) -> Mux6/24
  BatteryModelAdvanced/145(Cell_ocv25) -> Mux6/25
  BatteryModelAdvanced/146(Cell_ocv26) -> Mux6/26
  BatteryModelAdvanced/147(Cell_ocv27) -> Mux6/27
  BatteryModelAdvanced/148(Cell_ocv28) -> Mux6/28
  BatteryModelAdvanced/149(Cell_ocv29) -> Mux6/29
  BatteryModelAdvanced/150(Cell_ocv30) -> Mux6/30
  BatteryModelAdvanced/151(Cell_ocv31) -> Mux6/31
  BatteryModelAdvanced/152(Cell_ocv32) -> Mux6/32
  BatteryModelAdvanced/153(Cell_ocv33) -> Mux6/33
  BatteryModelAdvanced/154(Cell_ocv34) -> Mux6/34
  BatteryModelAdvanced/155(Cell_ocv35) -> Mux6/35
  BatteryModelAdvanced/156(Cell_ocv36) -> Mux6/36
  BatteryModelAdvanced/157(Cell_ocv37) -> Mux6/37
  BatteryModelAdvanced/158(Cell_ocv38) -> Mux6/38
  BatteryModelAdvanced/159(Cell_ocv39) -> Mux6/39
  BatteryModelAdvanced/160(Cell_ocv40) -> Mux6/40
  BatteryModelAdvanced/165(pack_soc) -> Unit Delay3/1
  BatteryModelAdvanced/164(pack_current) -> Unit Delay2/1
  BatteryModelAdvanced/163(vehicle_side_voltage) -> Unit Delay1/1
  BatteryModelAdvanced/162(pack_voltage) -> Unit Delay/1
  BatteryModelAdvanced/161(outlet_temperature) -> Unit Delay6/1
  Unit Delay6/1 -> outlet_temperature/1
  CB_cmds/1 -> Data Type Conversion6/1
  Data Type Conversion6/1 -> Demux/1
  Demux/1 -> BatteryModelAdvanced/1(cmd_1)
  Demux/2 -> BatteryModelAdvanced/2(cmd_2)
  Demux/3 -> BatteryModelAdvanced/3(cmd_3)
  Demux/4 -> BatteryModelAdvanced/4(cmd_4)
  Demux/5 -> BatteryModelAdvanced/5(cmd_5)
  Demux/6 -> BatteryModelAdvanced/6(cmd_6)
  Demux/7 -> BatteryModelAdvanced/7(cmd_7)
  Demux/8 -> BatteryModelAdvanced/8(cmd_8)
  Demux/9 -> BatteryModelAdvanced/9(cmd_9)
  Demux/10 -> BatteryModelAdvanced/10(cmd_10)
  Demux/11 -> BatteryModelAdvanced/11(cmd_11)
  Demux/12 -> BatteryModelAdvanced/12(cmd_12)
  Demux/13 -> BatteryModelAdvanced/13(cmd_13)
  Demux/14 -> BatteryModelAdvanced/14(cmd_14)
  Demux/15 -> BatteryModelAdvanced/15(cmd_15)
  Demux/16 -> BatteryModelAdvanced/16(cmd_16)
  Demux/17 -> BatteryModelAdvanced/17(cmd_17)
  Demux/18 -> BatteryModelAdvanced/18(cmd_18)
  Demux/19 -> BatteryModelAdvanced/19(cmd_19)
  Demux/20 -> BatteryModelAdvanced/20(cmd_20)
  Demux/21 -> BatteryModelAdvanced/21(cmd_21)
  Demux/22 -> BatteryModelAdvanced/22(cmd_22)
  Demux/23 -> BatteryModelAdvanced/23(cmd_23)
  Demux/24 -> BatteryModelAdvanced/24(cmd_24)
  Demux/25 -> BatteryModelAdvanced/25(cmd_25)
  Demux/26 -> BatteryModelAdvanced/26(cmd_26)
  Demux/27 -> BatteryModelAdvanced/27(cmd_27)
  Demux/28 -> BatteryModelAdvanced/28(cmd_28)
  Demux/29 -> BatteryModelAdvanced/29(cmd_29)
  Demux/30 -> BatteryModelAdvanced/30(cmd_30)
  Demux/31 -> BatteryModelAdvanced/31(cmd_31)
  Demux/32 -> BatteryModelAdvanced/32(cmd_32)
  Demux/33 -> BatteryModelAdvanced/33(cmd_33)
  Demux/34 -> BatteryModelAdvanced/34(cmd_34)
  Demux/35 -> BatteryModelAdvanced/35(cmd_35)
  Demux/36 -> BatteryModelAdvanced/36(cmd_36)
  Demux/37 -> BatteryModelAdvanced/37(cmd_37)
  Demux/38 -> BatteryModelAdvanced/38(cmd_38)
  Demux/39 -> BatteryModelAdvanced/39(cmd_39)
  Demux/40 -> BatteryModelAdvanced/40(cmd_40)
  pre_cc_cmd/1 -> Data Type Conversion1/1
  neg_cc_cmd/1 -> Data Type Conversion2/1
  chg_cc_cmd/1 -> Logical Operator/2, Data Type Conversion3/1
  fan_cmd/1 -> Data Type Conversion4/1
  cabin_temperature/1 -> Data Type Conversion5/1
  Data Type Conversion/1 -> BatteryModelAdvanced/41(main_cc_comd)
  Data Type Conversion1/1 -> BatteryModelAdvanced/42(pre_cc_cmd)
  Data Type Conversion2/1 -> BatteryModelAdvanced/43(neg_cc_cmd)
  Data Type Conversion3/1 -> BatteryModelAdvanced/44(chg_cc_cmd)
  Data Type Conversion4/1 -> BatteryModelAdvanced/45(fan_cmd)
  Data Type Conversion5/1 -> BatteryModelAdvanced/46(cabin_temp)
  Idischg_max/1 -> Unary Minus1/1
  Subsystem/1(input_I) -> Data Type Conversion9/1
  Data Type Conversion7/1 -> BatteryModelAdvanced/47(Ichg_max)
  Data Type Conversion8/1 -> BatteryModelAdvanced/48(Idischg_max)
  Data Type Conversion9/1 -> BatteryModelAdvanced/49(input_current)
  Data Type Conversion10/1 -> BatteryModelAdvanced/50(load_type)
  Unary Minus1/1 -> Data Type Conversion8/1
  main_cc_cmd/1 -> Logical Operator/1
  Logical Operator/1 -> Data Type Conversion/1
  Ichg_max/1 -> Data Type Conversion7/1, Subsystem/1(Ichg_max)
  From Workspace/1 -> Data Type Conversion10/1
